simulink model "linear_mpc"  (R2018b)
settings: Solver=VariableStepAuto  StartTime=0.0  StopTime=40.0  RelTol=1e-3
model workspace (MAT data in the model file):
  op_trim1 : opcond.OperatingReport (value not decoded)
  op_trim2 : opcond.OperatingReport (value not decoded)
  op_trim3 : opcond.OperatingReport (value not decoded)
undefined symbols (not defined in the file or in its folder): magnitude
libraries: mpclib x1, simulink x1
settings Model: Creator=Alberic  LastModifiedBy=Alberic
settings DataIOCC: ExternalInput=getinputstruct(op_trim1)  InitialState=getstatestruct(op_trim1)  LoadExternalInput=on  LoadInitialState=on

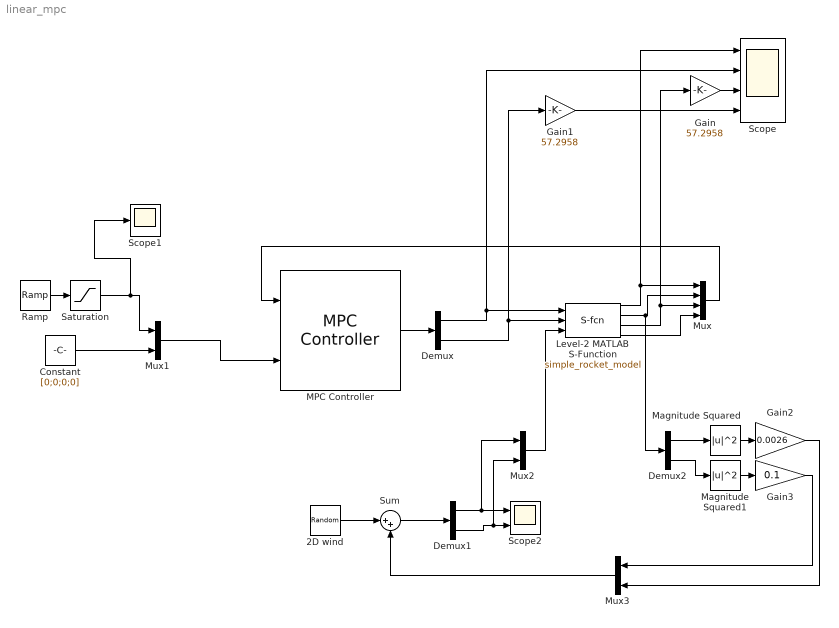
== system linear_mpc ==
  2D wind : RandomNumber  Mean=[0;0]  Variance=[5;1e1]  Seed=[1;2]  SampleTime=0.1
  Constant : Constant  Value=[0;0;0;0]
  Demux : Demux  Outputs=2
  Demux1 : Demux  Outputs=2
  Demux2 : Demux  Outputs=2
  Gain : Gain  Gain=57.2958
  Gain1 : Gain  Gain=57.2958
  Gain2 : Gain  Gain=0.0026
  Gain3 : Gain  Gain=0.1
  Level-2 MATLAB S-Function : M-S-Function  FunctionName=simple_rocket_model  Parameters=1, 0.083, 0.5
  MPC Controller : mpclib/MPC Controller  SCDEnableBlockLinearizationSpecification=on  mpcobj=mpc1  is_multiple=0  enable_value=0  return_u0=off  updateMPCinCallerWorkspace=on  md_inport=off  mv_inport=off  return_cost=off  return_mvseq=off  return_qpstatus=off  return_xseq=off  return_state=off  return_ovseq=off  state_inport=off  umin_inport=off  umax_inport=off  ymin_inport=off  ymax_inport=off  cc_inport=off  ywt_inport=off  uwt_inport=off  duwt_inport=off  rhoeps_inport=off  uref_inport=off  n_ts=0.1  n_p=20  n_mv=2  n_md=0  n_ud=2  n_mo=6  n_uo=0  BlockDataType=double  SampleTimeInherited=off  switch_inport=off
  Magnitude Squared : Math  Operator=magnitude^2  SaturateOnIntegerOverflow=on
  Magnitude Squared1 : Math  Operator=magnitude^2  SaturateOnIntegerOverflow=on
  Mux : Mux
  Mux1 : Mux  Inputs=2
  Mux2 : Mux  Inputs=2
  Mux3 : Mux  Inputs=2
  Ramp : simulink/Sources/Ramp  slope=[1;20]  start=[20;5]  InitialOutput=[0;2]
  Saturation : Saturate  UpperLimit=[10;50]  LowerLimit=0
  Scope : Scope  NumInputPorts=4
  Scope1 : Scope
  Scope2 : Scope  NumInputPorts=2
  Sum : Sum  Inputs=|++
  wires:
  Level-2 MATLAB S-Function/1 -> Scope/1, Mux/1
  Level-2 MATLAB S-Function/3 -> Mux/3, Gain/1
  Gain/1 -> Scope/3
  Gain1/1 -> Scope/4
  Mux/1 -> MPC Controller/1
  Constant/1 -> Mux1/2
  Ramp/1 -> Saturation/1
  Saturation/1 -> Scope1/1, Mux1/1
  Demux/1 -> Level-2 MATLAB S-Function/1, Scope/2
  Demux/2 -> Gain1/1, Level-2 MATLAB S-Function/2
  Demux1/1 -> Mux2/1, Scope2/1
  Demux1/2 -> Mux2/2, Scope2/2
  Level-2 MATLAB S-Function/2 -> Demux2/1, Mux/2
  Level-2 MATLAB S-Function/4 -> Mux/4
  Mux2/1 -> Level-2 MATLAB S-Function/3
  MPC Controller/1 -> Demux/1
  2D wind/1 -> Sum/1
  Demux2/1 -> Magnitude Squared/1
  Demux2/2 -> Magnitude Squared1/1
  Magnitude Squared/1 -> Gain2/1
  Magnitude Squared1/1 -> Gain3/1
  Gain2/1 -> Mux3/2
  Gain3/1 -> Mux3/1
  Mux3/1 -> Sum/2
  Sum/1 -> Demux1/1
  Mux1/1 -> MPC Controller/2
